simulink model "mytun"  (R2023b)
settings: Solver=FixedStepDiscrete  StartTime=0.0  StopTime=28  FixedStep=0.01  RelTol=1e-3
libraries: mobileRoboticsTrainingLib x12, robotmobilelib x1, slpidlib x1, simulink x1
settings Model: Creator=TRAN HOANG MINH NHUT  LastModifiedBy=TRAN HOANG MINH NHUT
settings RTWCC: GenCodeOnly=on

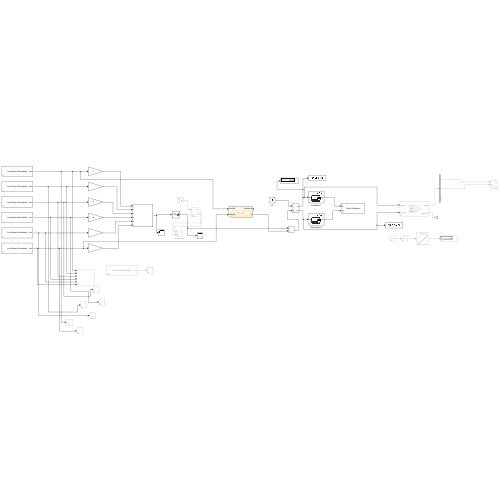
[thumbnail: Simulink's stored preview of the top-level diagram]
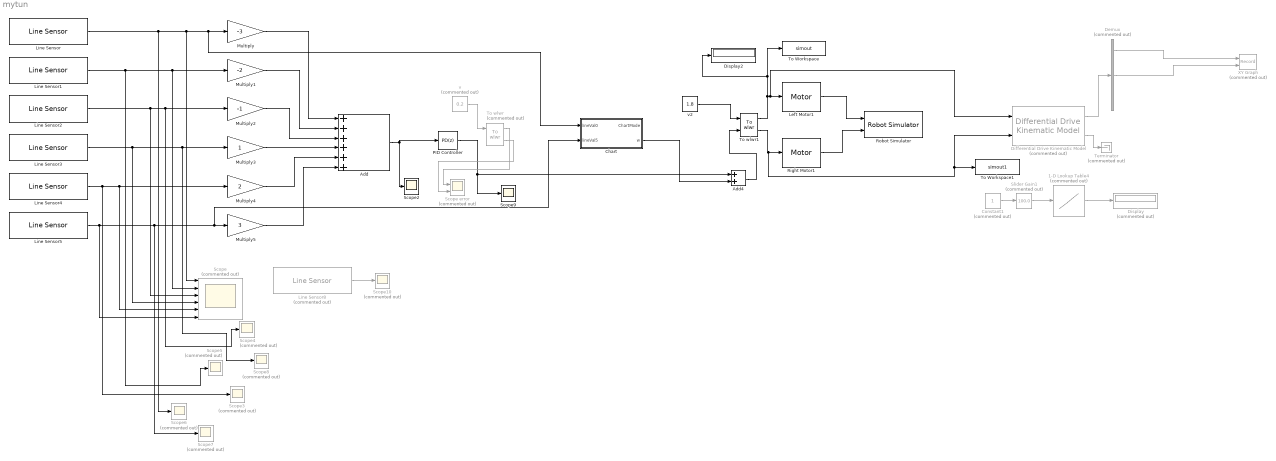
== system mytun ==
  1-D Lookup Table4 : Lookup_n-D  Commented=on  NumberOfTableDimensions=1  BreakpointsForDimension1=[0:1:100]  Table=[0:2:200]  ExtrapMethod=Clip  InternalRulePriority=Speed  RndMeth=Simplest
  Add : Sum  Inputs=++++++
  Add4 : Sum
  Chart : Stateflow chart  TreatAsAtomicUnit=on
  Constant1 : Constant  Commented=on
  Demux : Demux  Commented=on  Outputs=3
  Differential Drive Kinematic Model : robotmobilelib/Differential Drive Kinematic Model  Commented=on  VehicleInputs=Wheel Speeds  WheelRadius=0.0325  WheelSpeedRange=[-inf inf]  TrackWidth=0.026  InitialState=[0 ; 0; 0]  SimulateUsing=Interpreted execution
  Display : Display  Commented=on
  Display2 : Display
  Left Motor1 : mobileRoboticsTrainingLib/Motor  motorPlant=wheelMotorModel  sensorType=Speed
      settings: SourceProductName=Mobile Robotics Training Library
  Line Sensor : mobileRoboticsTrainingLib/Line Sensor  mapVariable=mapForSim  envVal=35  lineVal=315  sensOff=[0.2 0.0425]
      settings: SourceProductName=Mobile Robotics Training Library
  Line Sensor1 : mobileRoboticsTrainingLib/Line Sensor  mapVariable=mapForSim  envVal=35  lineVal=315  sensOff=[0.2 0.0255]
      settings: SourceProductName=Mobile Robotics Training Library
  Line Sensor2 : mobileRoboticsTrainingLib/Line Sensor  mapVariable=mapForSim  envVal=35  lineVal=315  sensOff=[0.2 0.0085]
      settings: SourceProductName=Mobile Robotics Training Library
  Line Sensor3 : mobileRoboticsTrainingLib/Line Sensor  mapVariable=mapForSim  envVal=35  lineVal=315  sensOff=[0.2 -0.0085]
      settings: SourceProductName=Mobile Robotics Training Library
  Line Sensor4 : mobileRoboticsTrainingLib/Line Sensor  mapVariable=mapForSim  envVal=35  lineVal=315  sensOff=[0.2 -0.0255]
      settings: SourceProductName=Mobile Robotics Training Library
  Line Sensor5 : mobileRoboticsTrainingLib/Line Sensor  mapVariable=mapForSim  envVal=35  lineVal=315  sensOff=[0.2 -0.0425]
      settings: SourceProductName=Mobile Robotics Training Library
  Line Sensor8 : mobileRoboticsTrainingLib/Line Sensor  Commented=on  mapVariable=mapForSim  envVal=35  lineVal=315  sensOff=[0 0]
      settings: SourceProductName=Mobile Robotics Training Library
  Multiply : Gain  Gain=-3
  Multiply1 : Gain  Gain=-2
  Multiply2 : Gain  Gain=-1
  Multiply3 : Gain
  Multiply4 : Gain  Gain=2
  Multiply5 : Gain  Gain=3
  PID Controller : slpidlib/PID Controller  Controller=PD  Form=Parallel  TimeDomain=Discrete-time  UseExternalTs=off  SampleTime=-1  IntegratorMethod=Forward Euler  FilterMethod=Forward Euler  ControllerParametersSource=internal  P=-0.004  I=500  UseKiTs=off  D=(1e-5)  N=100  UseFilter=on  TunerSelectOption=Transfer Function Based (PID Tuner App)  InitialConditionSource=internal  InitialConditionForIntegrator=0  InitialConditionForFilter=0  DifferentiatorICPrevScaledInput=0  ExternalReset=none  TrackingMode=off  Kt=1  LimitOutput=on  SatLimitsSource=internal  UpperSaturationLimit=4  LowerSaturationLimit=-4  LinearizeAsGain=on  AntiWindupMode=none  Kb=1  LimitIntegrator=off  UpperIntegratorSaturationLimit=inf  LowerIntegratorSaturationLimit=-inf  POutMin=[]  POutMax=[]  IOutMin=[]  IOutMax=[]  DOutMin=[]  DOutMax=[]  NOutMin=[]  NOutMax=[]  SumOutMin=[]  SumOutMax=[]  SaturationOutMin=[]  SaturationOutMax=[]  PParamMin=[]  PParamMax=[]  IParamMin=[]  IParamMax=[]  DParamMin=[]  DParamMax=[]  NParamMin=[]  NParamMax=[]  KbParamMin=[]  KbParamMax=[]  KtParamMin=[]  KtParamMax=[]  KbOutMin=[]  KbOutMax=[]  KtOutMin=[]  KtOutMax=[]  IntegratorOutMin=[]  IntegratorOutMax=[]  FilterOutMin=[]  FilterOutMax=[]  SumI1OutMin=[]  SumI1OutMax=[]  SumI2OutMin=[]  SumI2OutMax=[]  SumI3OutMin=[]  SumI3OutMax=[]  SumI4OutMin=[]  SumI4OutMax=[]  SumDOutMin=[]  SumDOutMax=[]  DifferentiatorOutMin=[]  DifferentiatorOutMax=[]  FilterDiffOutCoefMin=[]  FilterDiffOutCoefMax=[]  ReciprocalOutMin=[]  ReciprocalOutMax=[]  SumDenOutMin=[]  SumDenOutMax=[]  SumNumOutMin=[]  SumNumOutMax=[]  DivideOutMin=[]  DivideOutMax=[]  UdiffTsProdOutMin=[]  UdiffTsProdOutMax=[]  NTsProdOutMin=[]  NTsProdOutMax=[]  UintegralTsProdOutMin=[]  UintegralTsProdOutMax=[]  UngainTsProdOutMin=[]  UngainTsProdOutMax=[]  ClampingZeroOutDataTypeStr=Inherit: Inherit via back propagation  ClampingZeroOutMin=[]  ClampingZeroOutMax=[]  FilterDenConstantOutDataTypeStr=Inherit: Inherit via back propagation  FilterDenConstantOutMin=[]  FilterDenConstantOutMax=[]  PCopyOutDataTypeStr=Inherit: Inherit via back propagation  PCopyOutMin=[]  PCopyOutMax=[]  NCopyOutDataTypeStr=Inherit: Inherit via back propagation  NCopyOutMin=[]  NCopyOutMax=[]  IntegratorContinuousStateAttributes=''  IntegratorStateMustResolveToSignalObject=off  IntegratorRTWStateStorageClass=Auto  FilterContinuousStateAttributes=''  FilterStateMustResolveToSignalObject=off  FilterRTWStateStorageClass=Auto  ParallelPVariant=InternalParameters  IdealPVariant=Disabled  IVariant=Disabled  DVariant=InternalParameters  IntegratorVariant=Disabled  SatVariant=Enabled  AWVariant=Disabled  PCopyVariant=Disabled  TRVariant=Disabled  FdbkBlocksVariant=Forward  IdealPFdbkVariant=Disabled  SatFdbkVariant=Disabled  DerivativeFilterVariant=ForwardEulerFilter  NVariant=InternalParameters  NCopyVariant=Disabled  FilterICVariant=InternalICsFilter  IntegratorICVariant=Disabled  ExternalResetVariant=Disabled  TRSumVariant=Passthrough  SumFdbkVariant=Disabled  SumVariant=Sum_PD  TsampFilterVariant=InternalTs  TsampNgainVariant=Passthrough  TsampIntegralVariant=Disabled_SignalSpec  ExternalSaturationOutDataTypeStr=Inherit: Same as second input  InitialConditionSetting=Output
  Right Motor1 : mobileRoboticsTrainingLib/Motor  motorPlant=wheelMotorModel  sensorType=Speed
      settings: SourceProductName=Mobile Robotics Training Library
  Robot Simulator : mobileRoboticsTrainingLib/Robot Simulator  Priority=99  mapVar=mapForSim  startX=3.1341  startY=0.15079  startTheta=180  axleLength=axleLength  wheelR=wheelR
  Scope : Scope  Commented=on  NumInputPorts=6
  Scope error : Scope  Commented=on  NumInputPorts=2
  Scope{3..8,10} (7 alike) : Scope  Commented=on
  Scope2 : Scope
  Scope9 : Scope
  Slider Gain1 : simulink/Math Operations/Slider Gain  Commented=on  gain=100.0  low=0  high=100
  Terminator : Terminator  Commented=on
  To Workspace : ToWorkspace  VariableName=simout  SaveFormat=Structure  SampleTime=-1
  To Workspace1 : ToWorkspace  VariableName=simout1  SaveFormat=Structure  SampleTime=-1
  To wlwr : mobileRoboticsTrainingLib/To wlwr  Commented=on  axleLength=axleLength  wheelR=wheelR
  To wlwr1 : mobileRoboticsTrainingLib/To wlwr  axleLength=axleLength  wheelR=wheelR
  XY Graph : Record  Commented=on  FileSettingsInternal="{\"entries\":[{\"content\":{\"excelSettings\":{\"content\":{},\"type\":\"Streamout.ExcelSettings\"}},\"type\":\"Streamout.FileSettingStorage\",\"uuid\":\"\"}],\"packageUris\":[\"http:\\/\\/schema.mathworks.com\\/mf0\\/streamout_blocks\\/R2020a\"],\"version\":\"1.0\"}"  Layout=[1 1]  SignalsInternal="{\"entries\":[{\"content\":{},\"type\":\"RecordBlkView.InputSignals\",\"uuid\":\"\"}],\"packageUris\":[\"http:\\/\\/schema.mathworks.com\\/mf0\\/streamout_blocks\\/R2020a\"],\"version\":\"1.0\"}"  VisualizationBindings="{\"xyplotplugin\":{\"info\":[{\"series\":[],\"subplotID\":1}]}}"  CompatibilityTag=XY
  v : Constant  Commented=on  Value=0.2
  v2 : Constant  Value=1.8
  wires:
  PID Controller/1 -> Scope9/1, Add4/1
  Line Sensor/1 -> Scope/1, Chart/1(lineVal0), Multiply/1, Scope6/1
  v/1 -> To wlwr/1
  Line Sensor3/1 -> Scope/4, Scope8/1, Multiply3/1
  Line Sensor4/1 -> Scope3/1, Scope/5, Multiply4/1
  Line Sensor5/1 -> Scope/6, Scope7/1, Chart/2(lineVal5), Multiply5/1
  Multiply/1 -> Add/1
  Multiply1/1 -> Add/2
  Multiply2/1 -> Add/3
  Multiply3/1 -> Add/4
  Multiply4/1 -> Add/5
  Multiply5/1 -> Add/6
  Demux/2 -> XY Graph/2
  Demux/1 -> XY Graph/1
  To wlwr/1 -> Scope error/1
  To wlwr/2 -> Scope error/2
  v2/1 -> To wlwr1/1
  Add/1 -> Scope2/1, PID Controller/1
  Line Sensor1/1 -> Scope5/1, Scope/2, Multiply1/1
  Line Sensor2/1 -> Scope4/1, Multiply2/1, Scope/3
  To wlwr1/1 -> Display2/1, To Workspace/1, Differential Drive Kinematic Model/1, Left Motor1/1
  Left Motor1/1 -> Robot Simulator/1
  To wlwr1/2 -> To Workspace1/1, Differential Drive Kinematic Model/2, Right Motor1/1
  Right Motor1/1 -> Robot Simulator/2
  1-D Lookup Table4/1 -> Display/1
  Constant1/1 -> Slider Gain1/1
  Slider Gain1/1 -> 1-D Lookup Table4/1
  Chart/2(w) -> Add4/2
  Add4/1 -> To wlwr1/2
  Line Sensor8/1 -> Scope10/1
  Differential Drive Kinematic Model/1 -> Demux/1
  Differential Drive Kinematic Model/2 -> Terminator/1

== stateflow chart mytun/Chart ==
  state time_17
    w = 0
  state time_18
    w = -1
  (default) -> time_17
  time_17 -> time_18 : [lineVal0>200 && lineVal5>200]
  time_18 -> time_17
  data: ChartMode output Enum: ChartModeType; lineVal0 input; lineVal5 input; w output
